simulink model "vds"  (R2023b)
settings: Solver=ode1  StartTime=0.0  StopTime=6  FixedStep=0.001  RelTol=1e-3
values from neighbouring files (symbols this model uses):
  dist_cog_RA = 0.5    [pegasus_acc.m]
  long_acc = 2100    [pegasus_acc.m]
  m = m_base    (= 210)    [pegasus_acc.m]
  rear_front_split = 1    [pegasus_acc.m]
  track_FA = 1.5    [pegasus_acc.m]
  track_RA = 1.5    [pegasus_acc.m]
libraries: autolibshared x1
settings Model: Creator=eliasniepotter  LastModifiedBy=eliasniepotter

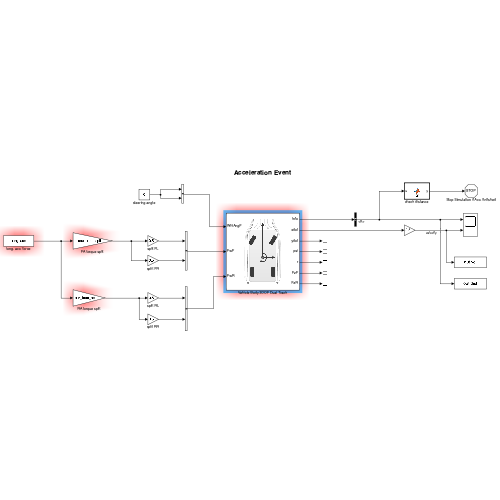
[thumbnail: Simulink's stored preview of the top-level diagram]
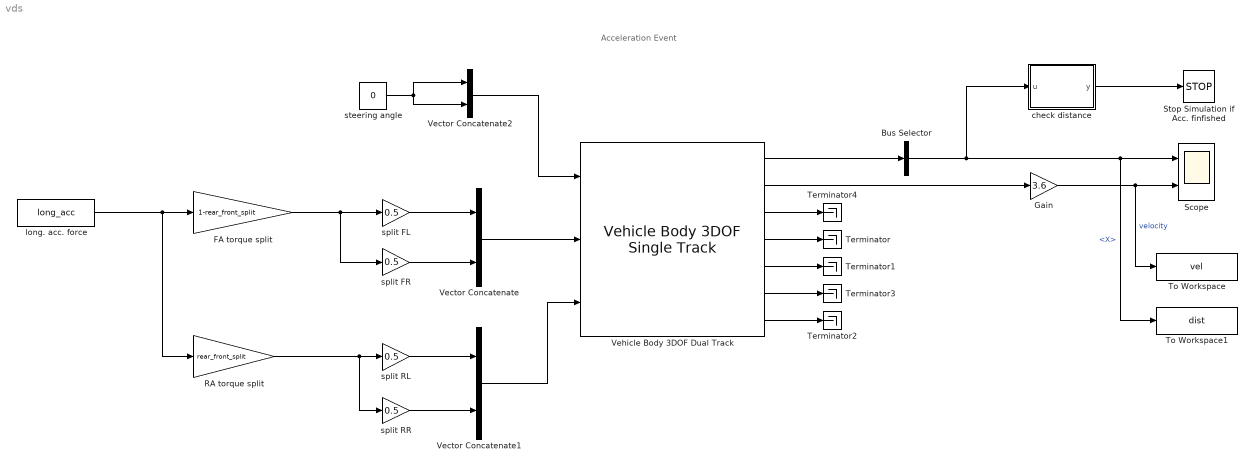
== system vds ==
  note: Acceleration Event
  Bus Selector : BusSelector  OutputSignals=InertFrm.Cg.Disp.X
  FA torque split : Gain  Gain=1-rear_front_split
  Gain : Gain  Gain=3.6
  RA torque split : Gain  Gain=rear_front_split
  Scope : Scope  NumInputPorts=2
  Stop Simulation if Acc. finfished : Stop
  Terminator{,1..4} (5 alike) : Terminator
  To Workspace : ToWorkspace  VariableName=vel  SampleTime=-1
  To Workspace1 : ToWorkspace  VariableName=dist  SampleTime=-1
  Vector Concatenate : Concatenate
  Vector Concatenate1 : Concatenate
  Vector Concatenate2 : Concatenate
  Vehicle Body 3DOF Dual Track : autolibshared/Vehicle Body 3DOF Single Track  trackMode=Dual  inputMode=External longitudinal forces  frontSteerMode=on  rearSteerMode=off  windMode=off  muMode=off  extFMode=off  extMMode=off  htchFMode=off  htchMMode=off  extXo=off  extpsio=off  extxdoto=off  extro=off  extYo=off  extTamb=off  extydoto=off  aMode=2  NF=2  NR=2  m=m  a=dist_cog_FA  b=dist_cog_RA  h=vert_dist_cog_axles  dh=1  hh=0.2  X_o=0  xdot_o=0  CalphaMode=off  sigmaMode=on  d=0  hl=0  w=[track_FA,track_RA]  Cy_f=12e3  Cy_r=11e3  sigma_f=.1  sigma_r=.1  alpha_f_brk=[-.1 .1]  Cy_f_data=[-9e3 9e3]  alpha_r_brk=[-.1 .1]  Cy_r_data=[-9e3 9e3]  Y_o=0  ydot_o=0  Izz=yaw_polar_inertia  psi_o=0  r_o=0  Af=aero_area  Cd=cd  Cl=cl  Cpm=.1  beta_w=[0 0.01:0.01:0.3]  Cs=[0:0.03:0.9]  Cym=[0 1e-6:0.01:0.3]  Pabs=101325  Tair=293  g=9.81  mu=1  xdot_tol=.001  Fznom=m*9.81/4  Fxtire_sat=7e4  Fytire_sat=7e4  longOff=0  latOff=0  vertOff=0  wrapAng=off
      settings: LibrarySourceBlock=vehdynlibeom/Vehicle Body 3DOF Dual Track
  check distance : MATLAB Function  TreatAsAtomicUnit=on
  long. acc. force : Constant  Value=long_acc
  split FL : Gain  Gain=0.5
  split FR : Gain  Gain=0.5
  split RL : Gain  Gain=0.5
  split RR : Gain  Gain=0.5
  steering angle : Constant  Value=0
  wires:
  long. acc. force/1 -> RA torque split/1, FA torque split/1
  Vehicle Body 3DOF Dual Track/2 -> Gain/1
  Vehicle Body 3DOF Dual Track/4 -> Terminator/1
  Vehicle Body 3DOF Dual Track/7 -> Terminator2/1
  Vehicle Body 3DOF Dual Track/5 -> Terminator1/1
  Vehicle Body 3DOF Dual Track/1 -> Bus Selector/1
  Bus Selector/1 -> check distance/1(u), To Workspace1/1, Scope/1  "<X>"
  Gain/1 -> To Workspace/1, Scope/2  "velocity"
  check distance/1(y) -> Stop Simulation if Acc. finfished/1
  Vehicle Body 3DOF Dual Track/6 -> Terminator3/1
  Vehicle Body 3DOF Dual Track/3 -> Terminator4/1
  FA torque split/1 -> split FR/1, split FL/1
  split FL/1 -> Vector Concatenate/1
  split FR/1 -> Vector Concatenate/2
  Vector Concatenate/1 -> Vehicle Body 3DOF Dual Track/2
  split RR/1 -> Vector Concatenate1/2
  RA torque split/1 -> split RR/1, split RL/1
  Vector Concatenate1/1 -> Vehicle Body 3DOF Dual Track/3
  split RL/1 -> Vector Concatenate1/1
  Vector Concatenate2/1 -> Vehicle Body 3DOF Dual Track/1
  steering angle/1 -> Vector Concatenate2/2, Vector Concatenate2/1

== matlab function vds/check distance ==
  data: u input; y output
function y = fcn(u)
    if u >= 75
        y = 1;
    else
        y = 0;
    end
